simulink model "B2B_MMC"  (R2018b)
settings: Solver=ode8  StartTime=0.0  StopTime=inf  FixedStep=10e-5  RelTol=1e-3
InitFcn:
  | Cd=100e-6;
  | Csm=3.3e-3;
  | L=4e-3;
  | R=0.1;
  | m=1;
  | N=9;
  | Nminus=N-1;
  | 
  | 
  | grid.vll_rms=10e3;
  | grid.f=50;
  | w=2*pi*grid.f;
  | grid.phase=0;
  | grid.va_peak=sqrt(2/3)*grid.vll_rms;
  | 
  | vd_ref=1.05*2*sqrt(2/3)*grid.vll_rms/m; % dc link voltage in pu
  | vsp_max=0.5*m*vd_ref; %phase voltage at phi=0
  | is_max=907;
  | Smax=3*grid.va_peak*is_max/2;
  | 
  | 
  | SCR= 100;  % INPUT SCR of grid at PCC = Ssc_grid/S_rated
  | %Calculated Grid impedance parameters
  | grid.L=grid.va_peak/(w*SCR*is_max); %Calculate Lg out of SRC and neglecting Rg
  | grid.R= w*grid.L/10;        % assume Rg = 10% of Xg [ohm];
  | grid.enable=1;
  | 
  | 
  | 
  | mmc1.load_percent=100;
  | mmc1.load_pf=0.9;
  | 
  | mmc2.load_percent=100;
  | mmc2.load_pf=0.9;
  | 
  | 
  | 
  | mmc1.occ_alpha = 2000;      % INPUT Desired BW output control test converter [rad/s]
  | mmc1.occ_alpha1 = 50;       % INPUT Desired BW of the resonant integrator [rad/s]
  | mmc1.occ_alpha_f = 1000;       % INPUT Desire BW of the VFF [rad/s]
  | 
  | mmc2.occ_alpha = 2000;      % INPUT Desired BW output control test converter [rad/s]
  | mmc2.occ_alpha1 = 50;       % INPUT Desired BW of the resonant integrator [rad/s}
  | mmc2.occ_alpha_f = 1000;       % INPUT Desire BW of the VFF [rad/s
  | 
  | 
  | mmc1.ccc_enable= 1; %INPUT enable ic controller
  | mmc1.ccc_time_enable= 0; %time when circ current control kicks in [s]
  | mmc1.ccc_alpha_cr= 30;  % INPUT BW of LPF for circ current to get the reference (dc value)[rad/s]
  | mmc1.ccc_Ra        = 10;       % INPUT Proportional gain of circ current control (R << Ra < Kp)
  | mmc1.ccc_alpha2 = 200;      % INPUT BW for circulating current test converter  (alpha_c < wgrid)[rad/s]
  | 
  | mmc2.ccc_enable= 1; %INPUT enable ic controller
  | mmc2.ccc_time_enable= 0; %time when circ current control kicks in [s]
  | mmc2.ccc_alpha_cr= 30;  % INPUT BW of LPF for circ current to get the reference (dc value)[rad/s]
  | mmc2.ccc_Ra        = 10;       % INPUT Proportional gain of circ current control (R << Ra < Kp)
  | mmc2.ccc_alpha2 = 200;      % INPUT BW for circulating current test converter  (alpha_c < wgrid)[rad/s]
  | 
  | 
  | mmc1.aec_enable_W= 1; %INPUT enable arm energy controller (Wsum and Wdelta)) at time_W_ctrl
  | mmc1.aec_time_enable_W= 0.8;  % INPUT time to enable W control [s]
  | mmc1.aec_time_Wsum_step = 3;  % INPUT Step time for Sum Energy Step [s]
  | mmc1.aec_WsumRefStep = -0.1;        % INPUT Sum Energy Step at time_SumEn_step [pu]
  | mmc1.aec_enable_Wsum_step  = 1; %INPUT enable Sum Energy step: WsumStep at time: time_WsumRef_step
  | mmc1.aec_alpha_W     = 50;         % INPUT Desired BW for W controler [rad/s]
  | 
  | mmc2.aec_enable_W= 1; %INPUT enable arm energy controller (Wsum and Wdelta)) at time_W_ctrl
  | mmc2.aec_time_enable_W= 0.8;  % INPUT time to enable W control [s]
  | mmc2.aec_time_Wsum_step = 3;  % INPUT Step time for Sum Energy Step [s]
  | mmc2.aec_WsumRefStep = -0.1;        % INPUT Sum Energy Step at time_SumEn_step [pu]
  | mmc2.aec_enable_Wsum_step  = 1; %INPUT enable Sum Energy step: WsumStep at time: time_WsumRef_step
  | mmc2.aec_alpha_W     = 50;         % INPUT Desired BW for W controler [rad/s]
  | 
  | 
  | 
  | mmc1.pll_alpha_b=2000;
  | mmc1.pll_kp=50;
  | mmc1.pll_ki=10;
  | 
  | mmc2.pll_alpha_b=2000;
  | mmc2.pll_kp=50;
  | mmc2.pll_ki=10;
  | 
  | 
  | mmc1.cvdc_alpha_d=50;
  | mmc1.cvdc_alpha_id=25;
  | mmc1.cvdc_enable=1;
  | 
  | mmc2.cvdc_alpha_d=50;
  | mmc2.cvdc_alpha_id=25;
  | mmc2.cvdc_enable=0;
libraries: powerlib x90, powerlib_meascontrol x10, rtlab x1, rtio_opalrt_op5142ex1 x1
(part 1 of 3)
settings Model: Creator=Silov  LastModifiedBy=Silov

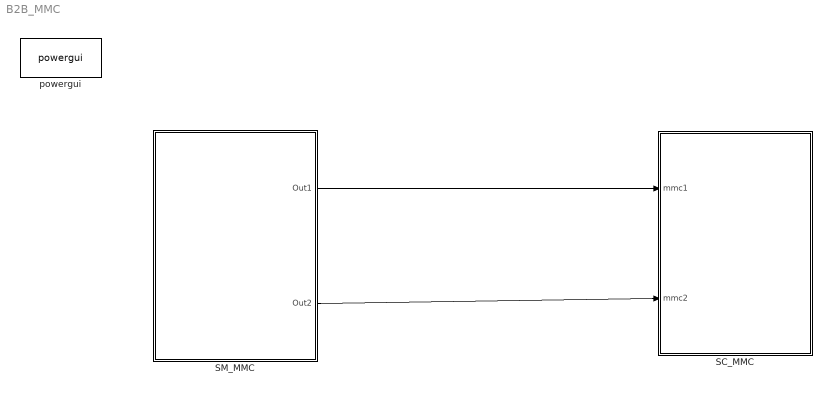
== system B2B_MMC ==
  SC_MMC : Subsystem
  SM_MMC : Subsystem
  powergui : powerlib/powergui  Priority=1  SimulationMode=Discrete  SampleTime=10e-5  frequency=60  Iterations=50  frequencyindice=0  Pbase=100e6  ErrMax=1e-4  UnitsV=kV  UnitsW=MW  buscounter=0  FunctionMessages=off  echomessages=off  EnableUseOfTLC=off  CurrentSourceSwitches=off  DisableSnubberDevices=off  DisableRonSwitches=off  DisableVfSwitches=off  DisplayEquations=off  SolverType=Tustin/Backward Euler (TBE)  Interpol=off  ExternalGateDelay=off  methode=off  Ts=100  x0status=blocks  SPID=on  SwTol=0  HookPort=off  RestoreLinks=warning  ResistiveCurrentMeasurement=off  Frange=[0:2:500]  Ylog=off  Xlog=on  ShowGrid=off  save=off  variable=ZData  structure=0  ZoomFFT=off  StartTime=0.0  cycles=1  DisplayStyle=1  fundamental=60  FreqAxis=off  MaxFrequency=1000  frequencyindicesteady=1  RmsSteady=1  display=off
  wires:
  SM_MMC/1(Out1) -> SC_MMC/1(mmc1)
  SM_MMC/2(Out2) -> SC_MMC/2(mmc2)

== system B2B_MMC/SC_MMC ==
  mmc1 : Inport
  mmc2 : Inport  Port=2
  Active power : Scope  NumInputPorts=2
  Demux : Demux  Outputs=3
  Demux1 : Demux  Outputs=3
  OpComm : rtlab/OpComm  nbport=2  groupe_acq=1  subsys_rate=0  st=0  Synchronization=on  Interpolation=on  Threshold=1.0  Missed_Data=off  Sim_Time=off  Samples=off  dynSigOut=off  from_console=0  warning_done=off  writeOpCommFile=off  Offset=off
  Reactive power : Scope  NumInputPorts=2
  "Voltage " : Scope  NumInputPorts=2
  wires:
  mmc1/1 -> OpComm/1
  mmc2/1 -> OpComm/2
  OpComm/1 -> Demux/1
  OpComm/2 -> Demux1/1
  Demux/1 -> "Voltage "/1
  Demux1/1 -> "Voltage "/2
  Demux/2 -> Active power/1
  Demux1/2 -> Active power/2
  Demux/3 -> Reactive power/1
  Demux1/3 -> Reactive power/2

== system B2B_MMC/SM_MMC ==
  MMC1 : Subsystem
  MMC2 : Subsystem
  OpCtrl OP5142EX1 : rtio_opalrt_op5142ex1/OpCtrl OP5142EX1  CtrlName='OP5142EX1 Ctrl'  boardid=0  BitstreamFilename=OP5142_1-EX-0000-2_2_6_61-16AO_32SelDIO_16AO_32SelDIO-01-01.bin  numconfig=-1  mode=Master  externalClock=off  decimRtsi=0  calibIO=off  SampleTime=0  loadinport=-1
  RSS Grid : Subsystem
  SSS Grid : Subsystem
  dc link impedance : powerlib/Elements/Series RLC Branch  LConnTagsString=__new0  RConnTagsString=__new0  BranchType=RL  Resistance=0.1  Inductance=0.0001  SetiL0=off  InitialCurrent=0  Capacitance=1e-6  Setx0=off  InitialVoltage=0  Measurements=None
  id : powerlib/Measurements/Current Measurement  PhasorSimulation=off  OutputType=Complex  PSBequivalent=0
  meter : powerlib/Measurements/Three-Phase V-I Measurement  VoltageMeasurement=phase-to-ground  SetLabelV=off  LabelV=Vabc  Vpu=off  VpuLL=off  CurrentMeasurement=no  SetLabelI=off  LabelI=Iabc  Ipu=off  Pbase=100e6  Vbase=500e3  OutputType=Complex  PhasorSimulation=off  PSBequivalent=0
  meter1 : powerlib/Measurements/Voltage Measurement  PhasorSimulation=off  OutputType=Complex  PSBequivalent=0
  meter2 : powerlib/Measurements/Three-Phase V-I Measurement  VoltageMeasurement=phase-to-ground  SetLabelV=off  LabelV=Vabc  Vpu=off  VpuLL=off  CurrentMeasurement=no  SetLabelI=off  LabelI=Iabc  Ipu=off  Pbase=100e6  Vbase=500e3  OutputType=Complex  PhasorSimulation=off  PSBequivalent=0
  meter3 : powerlib/Measurements/Voltage Measurement  PhasorSimulation=off  OutputType=Complex  PSBequivalent=0
  Out1 : Outport
  Out2 : Outport  Port=2
  tag scope: rss_vd=global, rss_vpcc=global, sss_id=global, sss_vd=global, sss_vpcc=global
  wires:
  meter1/1 -> [rss_vd]
  MMC1/1(mmc1) -> Out1/1
  meter/1 -> [sss_vpcc]
  meter2/1 -> [rss_vpcc]
  id/1 -> [sss_id]
  meter3/1 -> [sss_vd]
  MMC2/1(mmc2) -> Out2/1
  connections:
  meter1/LConn2 -- meter3/LConn2 -- MMC1/RConn2 -- MMC2/RConn2
  meter/RConn3 -- MMC1/LConn3
  meter/RConn2 -- MMC1/LConn2
  MMC1/RConn1 -- meter3/LConn1 -- id/LConn1
  MMC2/RConn1 -- dc link impedance/RConn1 -- meter1/LConn1
  MMC2/LConn3 -- meter2/RConn3
  meter/LConn2 -- SSS Grid/RConn2
  RSS Grid/RConn1 -- meter2/LConn1
  MMC2/LConn2 -- meter2/RConn2
  meter/RConn1 -- MMC1/LConn1
  meter2/LConn3 -- RSS Grid/RConn3
  MMC2/LConn1 -- meter2/RConn1
  id/RConn1 -- dc link impedance/LConn1
  SSS Grid/RConn3 -- meter/LConn3
  RSS Grid/RConn2 -- meter2/LConn2
  meter/LConn1 -- SSS Grid/RConn1

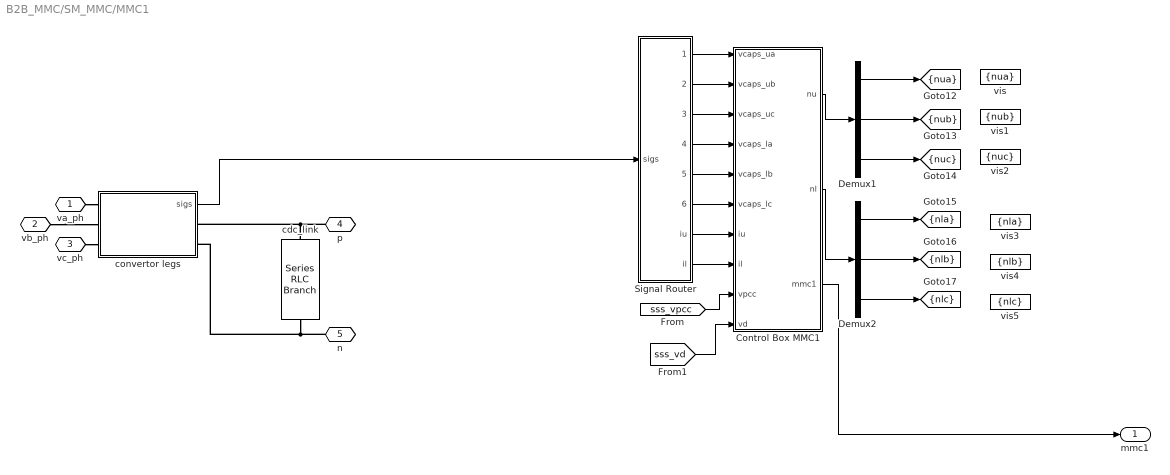
== system B2B_MMC/SM_MMC/MMC1 ==
  Control Box MMC1 : Subsystem  mask{N=N, R=R, L=L, Cd=Cd, Csm=Csm, vd_ref=vd_ref, is_max=is_max, vsp_max=vsp_max, Smax=Smax, occ_alpha=mmc1.occ_alpha, occ_alpha1=mmc1.occ_alpha1, occ_alpha_f=mmc1.occ_alpha_f, ccc_enable=mmc1.ccc_enable, ccc_enable_time=mmc1.ccc_time_enable, ccc_alpha_cr=mmc1.ccc_alpha_cr, ccc_Ra=mmc1.ccc_Ra, ccc_alpha2=mmc1.ccc_alpha2, aec_enable=mmc1.aec_enable_W, aec_enable_time=mmc1.aec_time_enable_W, aec_alpha_W=mmc1.aec_alpha_W, aec_enable_Wsum_step=mmc1.aec_enable_Wsum_step, aec_enable_time_Wsum_step=mmc1.aec_time_Wsum_step, aec_WsumRefStep=mmc1.aec_WsumRefStep, pll_alpha_b=mmc1.pll_alpha_b, pll_kp=mmc1.pll_kp, pll_ki=mmc1.pll_ki, load_percent=mmc1.load_percent, load_pf=mmc1.load_pf, cvdc_enable=mmc1.cvdc_enable, cvdc_alpha_d=mmc1.cvdc_alpha_d, cvdc_alpha_id=mmc1.cvdc_alpha_id}
      mask prompts: N "Number of Submodules"; R "Arm Resistance"; L "Arm Inductance (H)"; Cd "DC Link Capacitance (F)"; Csm "Submodule Capacitance (F)"; vd_ref "DC Link Reference Voltage  (V)"; is_max "Maximum AC Output Current (peak, A)"; vsp_max "Maximum AC Output Voltage (Peak, V)"; Smax "Maximum Apparent Power (VA)"; occ_alpha "Bandwidth, alpha (rad/s)"; occ_alpha1 "Bandwidth, integrator (rad/s)"; occ_alpha_f "Bandwidth for voltage feedforward (rad/s)"; ccc_enable "Enable"; ccc_enable_time "Time of Enable (s)"; ccc_alpha_cr "Bandwidth LPF for DC Reference (rad/s)"; ccc_Ra "Proportional Gain (Ra)"; ccc_alpha2 "Input bandwidth, alpha (rad/s)"; aec_enable "Enable"; aec_enable_time "Enable Time (s)"; aec_alpha_W "Bandwidth (rad/s)"; aec_enable_Wsum_step "Enable Wsum Step"; aec_enable_time_Wsum_step "Enable Wsum Step Time (s)"; aec_WsumRefStep "Step Change in Wsum (p.u.)"; pll_alpha_b "Bandwidth, alpha_b (rad/s)"; pll_kp "Proportional Gain (kp)"; pll_ki "Integral Gain"; load_percent "Percentage Load (%)"; load_pf "Power Factor"; cvdc_enable "Enable"; cvdc_alpha_d "alpha_d"; cvdc_alpha_id "alpha_id"
      mask init:
      | % Output Current Control
      | occ.alpha = occ_alpha;      % INPUT Desired BW output control test converter [rad/s]
      | occ.alpha1= occ_alpha1;       % INPUT Desired BW of the resonant integrator [rad/s}
      | occ.alpha_f = occ_alpha_f;       % INPUT Desire BW of the VFF [rad/s
      | occ.Kp   = occ_alpha*(L/2); % Proportional gain PR conrtoller for output currnet
      | occ.K1   = 2*occ_alpha1*occ.Kp; % Integral gain PI conrtoller for output currnet
      | 
      | % Ciculating current controller
      | ccc.alpha_cr= ccc_alpha_cr;  % INPUT BW of LPF for circ current to get the reference (dc value)[rad/s]
      | ccc.enable_int_ctrl= ccc_enable; %INPUT enable ic controller
      | ccc.time_enable_int_ctrl= ccc_enable_time; %time when circ current control kicks in [s]
      | ccc.Ra        = ccc_Ra;       % INPUT Proportional gain of circ current control (R << Ra < Kp)
      | ccc.alpha2 = ccc_alpha2;      % INPUT BW for circulating current test converter  (alpha_c < wgrid)[rad/s]
      | ccc.K2     = 2*ccc_alpha2;% integral gain for resonant controller for ic for h=2
      | ccc.K1     = ccc.K2;    % integral gain for resonant controller for ic for h=1 (same BW as h=2)
      | ccc.K0     = ccc.K2/10; % integral gain for integrator (alpha0_cc = alfa2_cc/100 << alpha2_cc)
      | 
      | %% Arm Energy Controller
      | aec.enable_W_ctrl= aec_enable; %INPUT enable arm energy controller (Wsum and Wdelta)) at time_W_ctrl
      | aec.time_enable_W_ctrl= aec_enable_time;  % INPUT time to enable W control [s]
      | 
      | WsumRef   = (Csm/N)*vd_ref^2;  % Sum Energy reference [J]
      | aec.alpha_W     = aec_alpha_W;         % INPUT Desired BW for W controler [rad/s]
      | aec.Kp_Wsum     = aec.alpha_W/vd_ref; % Kp*Vd = alpha_Wsum
      | aec.Kp_Wdelta   = aec.alpha_W/vsp_max; % Kp*Vsmax = alpha_Wdelta
      | 
      | aec.time_WsumRef_step = aec_enable_time_Wsum_step;  % INPUT Step time for Sum Energy Step [s]
      | aec.WsumRefStep = aec_WsumRefStep;        % INPUT Sum Energy Step at time_SumEn_step [pu]
      | aec.enable_Wsum_step  = aec_enable_Wsum_step; %INPUT enable Sum Energy step: WsumStep at time: time_WsumRef_step
      | 
      | % PLL Parameters
      | pll.alpha_b=pll_alpha_b;
      | pll.kp=pll_kp;
      | pll.ki=pll_ki;
      | 
      | % Power Control
      | load.percent=load_percent/100;
      | load.phi=acos(load_pf); % It seems that if load.phi is positive then i am injecting reactive power in the grid
      | 
      | % DC Voltage Control variable passes
      | 
      | cvdc.alpha_d=cvdc_alpha_d;
      | cvdc.alpha_id=cvdc_alpha_id;
      | cvdc.enable=cvdc_enable;
      mask DialogControl Parameters Prompt: MMC 1
      mask DialogControl Container7 Prompt: Parameters
      mask DialogControl Design Prompt: Converter Boundaries
      mask DialogControl Container12 Prompt: Current Controllers
      mask DialogControl Container21 Prompt: Output Current
      mask DialogControl Container14 Prompt: Circulating Current
      mask DialogControl Container15 Prompt: Arm Energy
      mask DialogControl Container23 Prompt: Higher Level Control
      mask DialogControl Container22 Prompt: PLL
      mask DialogControl Container20 Prompt: Active and Reactive Powers
      mask DialogControl Container9 Prompt: DC Voltage Control
  Demux1 : Demux  Outputs=3
  Demux2 : Demux  Outputs=3
  Signal Router : Subsystem
  cdc_link : powerlib/Elements/Series RLC Branch  LConnTagsString=__new0  RConnTagsString=__new0  BranchType=C  Resistance=1  Inductance=1e-3  SetiL0=off  InitialCurrent=0  Capacitance=Cd  Setx0=on  InitialVoltage=vd_ref  Measurements=None
  convertor legs : Subsystem
  vis : GotoTagVisibility  GotoTag=nua
  vis1 : GotoTagVisibility  GotoTag=nub
  vis2 : GotoTagVisibility  GotoTag=nuc
  vis3 : GotoTagVisibility  GotoTag=nla
  vis4 : GotoTagVisibility  GotoTag=nlb
  vis5 : GotoTagVisibility  GotoTag=nlc
  va_ph : PMIOPort  Side=Left
  vb_ph : PMIOPort  Port=2  Side=Left
  vc_ph : PMIOPort  Port=3  Side=Left
  p : PMIOPort  Port=4  Side=Right
  n : PMIOPort  Port=5  Side=Right
  mmc1 : Outport
  tag scope: nla=scoped, nlb=scoped, nlc=scoped, nua=scoped, nub=scoped, nuc=scoped
  wires:
  convertor legs/1(sigs) -> Signal Router/1(sigs)
  Signal Router/1(vc_ua) -> Control Box MMC1/1(vcaps_ua)
  Signal Router/2(vc_ub) -> Control Box MMC1/2(vcaps_ub)
  Signal Router/3(vc_uc) -> Control Box MMC1/3(vcaps_uc)
  Signal Router/4(vc_la) -> Control Box MMC1/4(vcaps_la)
  Signal Router/5(vc_lb) -> Control Box MMC1/5(vcaps_lb)
  Signal Router/6(vc_lc) -> Control Box MMC1/6(vcaps_lc)
  Signal Router/7(iu) -> Control Box MMC1/7(iu)
  Signal Router/8(il) -> Control Box MMC1/8(il)
  Demux2/1 -> [nla]
  Demux2/3 -> [nlc]
  Demux2/2 -> [nlb]
  Control Box MMC1/2(nl) -> Demux2/1
  Demux1/1 -> [nua]
  Demux1/3 -> [nuc]
  Demux1/2 -> [nub]
  Control Box MMC1/1(nu) -> Demux1/1
  [sss_vpcc] -> Control Box MMC1/9(vpcc)
  [sss_vd] -> Control Box MMC1/10(vd)
  Control Box MMC1/3(mmc1) -> mmc1/1
  connections:
  cdc_link/LConn1 -- p/RConn1 -- convertor legs/RConn1
  cdc_link/RConn1 -- n/RConn1 -- convertor legs/RConn2
  va_ph/RConn1 -- convertor legs/LConn1
  vb_ph/RConn1 -- convertor legs/LConn2
  vc_ph/RConn1 -- convertor legs/LConn3

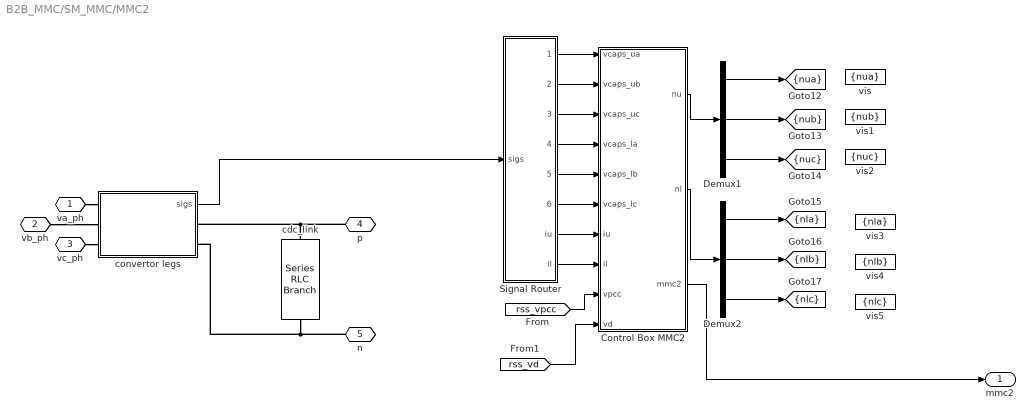
== system B2B_MMC/SM_MMC/MMC2 ==
  Control Box MMC2 : Subsystem  mask{N=N, R=R, L=L, Cd=Cd, Csm=Csm, vd_ref=vd_ref, is_max=is_max, vsp_max=vsp_max, Smax=Smax, occ_alpha=mmc2.occ_alpha, occ_alpha1=mmc2.occ_alpha1, occ_alpha_f=mmc2.occ_alpha_f, ccc_enable=mmc2.ccc_enable, ccc_enable_time=mmc2.ccc_time_enable, ccc_alpha_cr=mmc2.ccc_alpha_cr, ccc_Ra=mmc2.ccc_Ra, ccc_alpha2=mmc2.ccc_alpha2, aec_enable=mmc2.aec_enable_W, aec_enable_time=mmc2.aec_time_enable_W, aec_alpha_W=mmc2.aec_alpha_W, aec_enable_Wsum_step=mmc2.aec_enable_Wsum_step, aec_enable_time_Wsum_step=mmc2.aec_time_Wsum_step, aec_WsumRefStep=mmc2.aec_WsumRefStep, pll_alpha_b=mmc2.pll_alpha_b, pll_kp=mmc2.pll_kp, pll_ki=mmc2.pll_ki, load_percent=mmc2.load_percent, load_pf=mmc2.load_pf, cvdc_enable=mmc2.cvdc_enable, cvdc_alpha_d=mmc2.cvdc_alpha_d, cvdc_alpha_id=mmc2.cvdc_alpha_id}
      mask prompts: N "Number of Submodules"; R "Arm Resistance"; L "Arm Inductance (H)"; Cd "DC Link Capacitance (F)"; Csm "Submodule Capacitance (F)"; vd_ref "DC Link Reference Voltage  (V)"; is_max "Maximum AC Output Current (peak, A)"; vsp_max "Maximum AC Output Voltage (Peak, V)"; Smax "Maximum Apparent Power (VA)"; occ_alpha "Bandwidth, alpha (rad/s)"; occ_alpha1 "Bandwidth, integrator (rad/s)"; occ_alpha_f "Bandwidth for voltage feedforward (rad/s)"; ccc_enable "Enable"; ccc_enable_time "Time of Enable (s)"; ccc_alpha_cr "Bandwidth LPF for DC Reference (rad/s)"; ccc_Ra "Proportional Gain (Ra)"; ccc_alpha2 "Input bandwidth, alpha (rad/s)"; aec_enable "Enable"; aec_enable_time "Enable Time (s)"; aec_alpha_W "Bandwidth (rad/s)"; aec_enable_Wsum_step "Enable Wsum Step"; aec_enable_time_Wsum_step "Enable Wsum Step Time (s)"; aec_WsumRefStep "Step Change in Wsum (p.u.)"; pll_alpha_b "Bandwidth, alpha_b (rad/s)"; pll_kp "Proportional Gain (kp)"; pll_ki "Integral Gain"; load_percent "Percentage Load (%)"; load_pf "Power Factor"; cvdc_enable "Enable"; cvdc_alpha_d "alpha_d"; cvdc_alpha_id "alpha_id"
      mask init: same as B2B_MMC/SM_MMC/MMC1/Control Box MMC1
      mask DialogControl Parameters Prompt: MMC 1
      mask DialogControl Container7 Prompt: Parameters
      mask DialogControl Design Prompt: Converter Boundaries
      mask DialogControl Container12 Prompt: Current Controllers
      mask DialogControl Container21 Prompt: Output Current
      mask DialogControl Container14 Prompt: Circulating Current
      mask DialogControl Container15 Prompt: Arm Energy
      mask DialogControl Container23 Prompt: Higher Level Control
      mask DialogControl Container22 Prompt: PLL
      mask DialogControl Container20 Prompt: Active and Reactive Powers
      mask DialogControl Container9 Prompt: DC Voltage Control
  Demux1 : Demux  Outputs=3
  Demux2 : Demux  Outputs=3
  Signal Router : Subsystem
  cdc_link : powerlib/Elements/Series RLC Branch  LConnTagsString=__new0  RConnTagsString=__new0  BranchType=C  Resistance=1  Inductance=1e-3  SetiL0=off  InitialCurrent=0  Capacitance=Cd  Setx0=on  InitialVoltage=vd_ref  Measurements=None
  convertor legs : Subsystem
  vis : GotoTagVisibility  GotoTag=nua
  vis1 : GotoTagVisibility  GotoTag=nub
  vis2 : GotoTagVisibility  GotoTag=nuc
  vis3 : GotoTagVisibility  GotoTag=nla
  vis4 : GotoTagVisibility  GotoTag=nlb
  vis5 : GotoTagVisibility  GotoTag=nlc
  va_ph : PMIOPort  Side=Left
  vb_ph : PMIOPort  Port=2  Side=Left
  vc_ph : PMIOPort  Port=3  Side=Left
  p : PMIOPort  Port=4  Side=Right
  n : PMIOPort  Port=5  Side=Right
  mmc2 : Outport
  tag scope: nla=scoped, nlb=scoped, nlc=scoped, nua=scoped, nub=scoped, nuc=scoped
  wires:
  convertor legs/1(sigs) -> Signal Router/1(sigs)
  Signal Router/1(vc_ua) -> Control Box MMC2/1(vcaps_ua)
  Signal Router/2(vc_ub) -> Control Box MMC2/2(vcaps_ub)
  Signal Router/3(vc_uc) -> Control Box MMC2/3(vcaps_uc)
  Signal Router/4(vc_la) -> Control Box MMC2/4(vcaps_la)
  Signal Router/5(vc_lb) -> Control Box MMC2/5(vcaps_lb)
  Signal Router/6(vc_lc) -> Control Box MMC2/6(vcaps_lc)
  Signal Router/7(iu) -> Control Box MMC2/7(iu)
  Signal Router/8(il) -> Control Box MMC2/8(il)
  Demux2/1 -> [nla]
  Demux2/3 -> [nlc]
  Demux2/2 -> [nlb]
  Control Box MMC2/2(nl) -> Demux2/1
  Demux1/1 -> [nua]
  Demux1/3 -> [nuc]
  Demux1/2 -> [nub]
  Control Box MMC2/1(nu) -> Demux1/1
  [rss_vpcc] -> Control Box MMC2/9(vpcc)
  [rss_vd] -> Control Box MMC2/10(vd)
  Control Box MMC2/3(mmc2) -> mmc2/1
  connections:
  cdc_link/LConn1 -- convertor legs/RConn1 -- p/RConn1
  cdc_link/RConn1 -- convertor legs/RConn2 -- n/RConn1
  va_ph/RConn1 -- convertor legs/LConn1
  vb_ph/RConn1 -- convertor legs/LConn2
  vc_ph/RConn1 -- convertor legs/LConn3

== system B2B_MMC/SM_MMC/RSS Grid ==
  Three-Phase Series RLC Branch : powerlib/Elements/Three-Phase Series RLC Branch  LConnTagsString=A|B|C  RConnTagsString=A|B|C  BranchType=RL  Resistance=grid.R  Inductance=grid.L  Capacitance=1e-6  Measurements=None
  grid voltage : Subsystem
  va_ph : PMIOPort  Side=Right
  vb_ph : PMIOPort  Port=2  Side=Right
  vc_ph : PMIOPort  Port=3  Side=Right
  connections:
  grid voltage/RConn1 -- Three-Phase Series RLC Branch/LConn1
  grid voltage/RConn2 -- Three-Phase Series RLC Branch/LConn2
  grid voltage/RConn3 -- Three-Phase Series RLC Branch/LConn3
  va_ph/RConn1 -- Three-Phase Series RLC Branch/RConn1
  Three-Phase Series RLC Branch/RConn2 -- vb_ph/RConn1
  vc_ph/RConn1 -- Three-Phase Series RLC Branch/RConn3

== system B2B_MMC/SM_MMC/SSS Grid ==
  Three-Phase Series RLC Branch : powerlib/Elements/Three-Phase Series RLC Branch  LConnTagsString=A|B|C  RConnTagsString=A|B|C  BranchType=RL  Resistance=grid.R  Inductance=grid.L  Capacitance=1e-6  Measurements=None
  grid voltage : Subsystem
  va_ph : PMIOPort  Side=Right
  vb_ph : PMIOPort  Port=2  Side=Right
  vc_ph : PMIOPort  Port=3  Side=Right
  connections:
  grid voltage/RConn1 -- Three-Phase Series RLC Branch/LConn1
  grid voltage/RConn2 -- Three-Phase Series RLC Branch/LConn2
  grid voltage/RConn3 -- Three-Phase Series RLC Branch/LConn3
  va_ph/RConn1 -- Three-Phase Series RLC Branch/RConn1
  Three-Phase Series RLC Branch/RConn2 -- vb_ph/RConn1
  vc_ph/RConn1 -- Three-Phase Series RLC Branch/RConn3

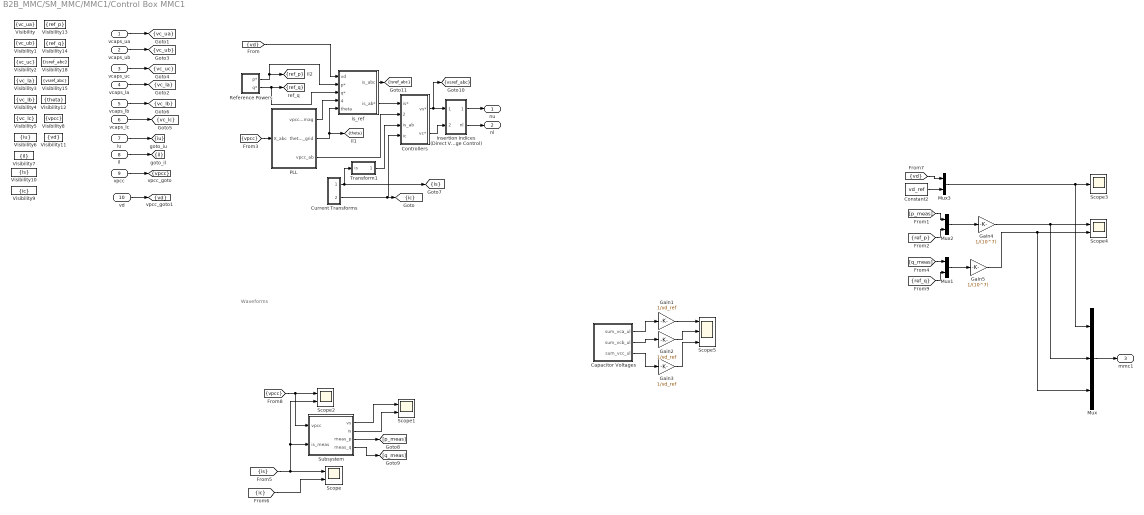
== system B2B_MMC/SM_MMC/MMC1/Control Box MMC1 ==
  note: Waveforms
  vcaps_ua : Inport
  vcaps_ub : Inport  Port=2
  vcaps_uc : Inport  Port=3
  vcaps_la : Inport  Port=4
  vcaps_lb : Inport  Port=5
  vcaps_lc : Inport  Port=6
  iu : Inport  Port=7
  il : Inport  Port=8
  vpcc : Inport  Port=9
  vd : Inport  Port=10
  Capacitor Voltages : Subsystem
  Constant2 : Constant  Value=vd_ref
  Controllers : Subsystem
  Current Transforms : Subsystem
  Gain1 : Gain  Gain=1/vd_ref
  Gain2 : Gain  Gain=1/vd_ref
  Gain3 : Gain  Gain=1/vd_ref
  Gain4 : Gain  Gain=1/(10^7)
  Gain5 : Gain  Gain=1/(10^7)
  Insertion Indices (Direct Voltage Control) : Subsystem
  Mux : Mux  Inputs=3
  Mux1 : Mux  Inputs=2
  Mux2 : Mux  Inputs=2
  Mux3 : Mux  Inputs=2
  PLL : Subsystem
  Reference Powers : Subsystem
  Scope{,1..2,4} (4 alike) : Scope  NumInputPorts=2
  Scope3 : Scope
  Scope5 : Scope  NumInputPorts=3
  Subsystem : Subsystem
  Transform1 : Subsystem
  Visibility : GotoTagVisibility  GotoTag=vc_ua
  Visibility1 : GotoTagVisibility  GotoTag=vc_ub
  Visibility10 : GotoTagVisibility  GotoTag=is
  Visibility11 : GotoTagVisibility  GotoTag=vd
  Visibility12 : GotoTagVisibility  GotoTag=theta
  Visibility13 : GotoTagVisibility  GotoTag=ref_p
  Visibility14 : GotoTagVisibility  GotoTag=ref_q
  Visibility15 : GotoTagVisibility  GotoTag=vsref_abc
  Visibility18 : GotoTagVisibility  GotoTag=isref_abc
  Visibility2 : GotoTagVisibility  GotoTag=vc_uc
  Visibility3 : GotoTagVisibility  GotoTag=vc_la
  Visibility4 : GotoTagVisibility  GotoTag=vc_lb
  Visibility5 : GotoTagVisibility  GotoTag=vc_lc
  Visibility6 : GotoTagVisibility  GotoTag=iu
  Visibility7 : GotoTagVisibility  GotoTag=il
  Visibility8 : GotoTagVisibility  GotoTag=vpcc
  Visibility9 : GotoTagVisibility  GotoTag=ic
  is_ref : Subsystem
  nu : Outport
  nl : Outport  Port=2
  mmc1 : Outport  Port=3
  tag scope: ic=scoped, il=scoped, is=scoped, isref_abc=scoped, iu=scoped, ref_p=scoped, ref_q=scoped, theta=scoped, vc_la=scoped, vc_lb=scoped, vc_lc=scoped, vc_ua=scoped, vc_ub=scoped, vc_uc=scoped, vd=scoped, vpcc=scoped, vsref_abc=scoped
  wires:
  Controllers/2(vc*) -> Insertion Indices (Direct Voltage Control)/2(vc*)
  Current Transforms/1(is) -> [is], Transform1/1(is)
  Reference Powers/2(q*) -> is_ref/3(q*), [ref_q]
  Transform1/1(is_ab) -> Controllers/3(is_ab)
  Controllers/1(vs*) -> [vsref_abc], Insertion Indices (Direct Voltage Control)/1(vs*)
  PLL/3(vpcc_ab) -> Controllers/2(vpcc_ab)
  is_ref/2(is_ab*) -> Controllers/1(is*)
  Current Transforms/2(ic) -> Controllers/4(ic), [ic]
  [vpcc] -> PLL/1(X_abc)
  is_ref/1(is_abc) -> [isref_abc]
  Reference Powers/1(p*) -> is_ref/2(p*), [ref_p]
  PLL/2(theta_grid) -> is_ref/5(theta), [theta]
  PLL/1(vpcc_mag) -> is_ref/4(vpll_mag)
  vcaps_ua/1 -> [vc_ua]
  vcaps_ub/1 -> [vc_ub]
  vcaps_uc/1 -> [vc_uc]
  iu/1 -> [iu]
  il/1 -> [il]
  vpcc/1 -> [vpcc]
  vcaps_la/1 -> [vc_la]
  vcaps_lb/1 -> [vc_lb]
  vcaps_lc/1 -> [vc_lc]
  Insertion Indices (Direct Voltage Control)/1(nu) -> nu/1
  Insertion Indices (Direct Voltage Control)/2(nl) -> nl/1
  vd/1 -> [vd]
  [vd] -> is_ref/1(vd)
  Mux3/1 -> Mux/1, Scope3/1
  Constant2/1 -> Mux3/2
  [vd] -> Mux3/1
  Subsystem/4(meas_q) -> [q_meas]
  Subsystem/3(meas_p) -> [p_meas]
  [is] -> Scope/1, Scope2/2, Subsystem/2(is_meas)
  [ic] -> Scope/2
  Capacitor Voltages/3(sum_vcc_ul) -> Gain3/1
  Capacitor Voltages/2(sum_vcb_ul) -> Gain2/1
  Capacitor Voltages/1(sum_vca_ul) -> Gain1/1
  Gain1/1 -> Scope5/1
  Gain2/1 -> Scope5/2
  Gain3/1 -> Scope5/3
  Gain5/1 -> Mux/3, Scope4/2
  Mux1/1 -> Gain5/1
  Gain4/1 -> Mux/2, Scope4/1
  Mux2/1 -> Gain4/1
  [q_meas] -> Mux1/1
  [ref_q] -> Mux1/2
  [p_meas] -> Mux2/1
  [ref_p] -> Mux2/2
  Subsystem/2(is) -> Scope1/2
  Subsystem/1(vs) -> Scope1/1
  [vpcc] -> Scope2/1, Subsystem/1(vpcc)
  Mux/1 -> mmc1/1

== system B2B_MMC/SM_MMC/MMC1/Signal Router ==
  sigs : Inport
  Demux : Demux  Outputs=12
  Mux : Mux  Inputs=3
  Mux1 : Mux  Inputs=3
  vc_ua : Outport
  vc_ub : Outport  Port=2
  vc_uc : Outport  Port=3
  vc_la : Outport  Port=4
  vc_lb : Outport  Port=5
  vc_lc : Outport  Port=6
  iu : Outport  Port=7
  il : Outport  Port=8
  wires:
  Demux/9 -> vc_uc/1
  Demux/1 -> Mux/1
  Demux/8 -> vc_ub/1
  Demux/7 -> vc_ua/1
  Demux/12 -> vc_lc/1
  Demux/3 -> Mux/3
  Demux/6 -> Mux1/3
  Demux/5 -> Mux1/2
  Mux1/1 -> il/1
  Demux/4 -> Mux1/1
  Demux/11 -> vc_lb/1
  sigs/1 -> Demux/1
  Mux/1 -> iu/1
  Demux/2 -> Mux/2
  Demux/10 -> vc_la/1

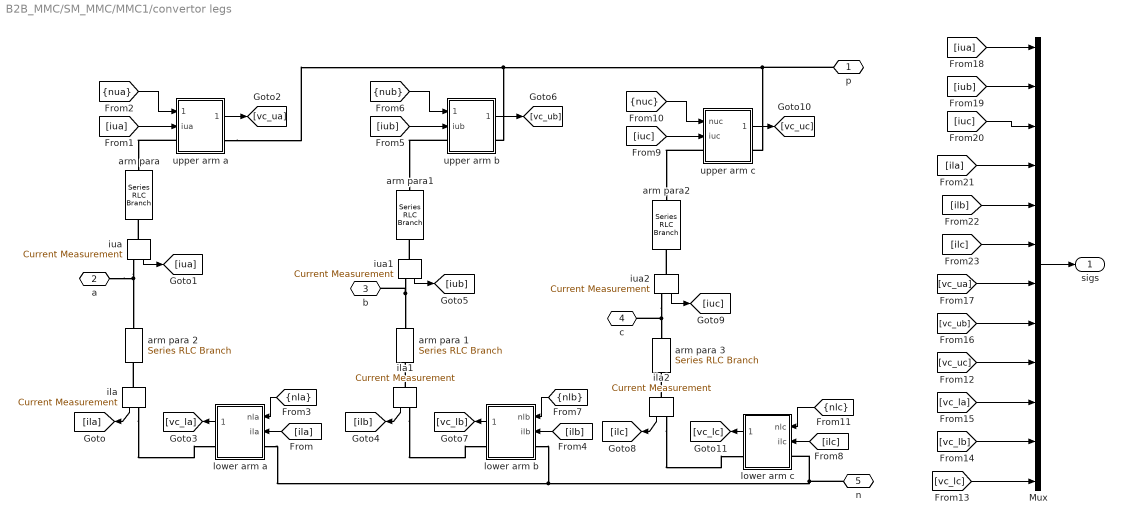
== system B2B_MMC/SM_MMC/MMC1/convertor legs ==
  Mux : Mux  Inputs=12
  arm para : powerlib/Elements/Series RLC Branch  LConnTagsString=__new0  RConnTagsString=__new0  BranchType=RL  Resistance=R  Inductance=L  SetiL0=off  InitialCurrent=0  Capacitance=1e-6  Setx0=off  InitialVoltage=0  Measurements=None
  arm para 1 : powerlib/Elements/Series RLC Branch  LConnTagsString=__new0  RConnTagsString=__new0  BranchType=RL  Resistance=R  Inductance=L  SetiL0=off  InitialCurrent=0  Capacitance=1e-6  Setx0=off  InitialVoltage=0  Measurements=None
  arm para 2 : powerlib/Elements/Series RLC Branch  LConnTagsString=__new0  RConnTagsString=__new0  BranchType=RL  Resistance=R  Inductance=L  SetiL0=off  InitialCurrent=0  Capacitance=1e-6  Setx0=off  InitialVoltage=0  Measurements=None
  arm para 3 : powerlib/Elements/Series RLC Branch  LConnTagsString=__new0  RConnTagsString=__new0  BranchType=RL  Resistance=R  Inductance=L  SetiL0=off  InitialCurrent=0  Capacitance=1e-6  Setx0=off  InitialVoltage=0  Measurements=None
  arm para1 : powerlib/Elements/Series RLC Branch  LConnTagsString=__new0  RConnTagsString=__new0  BranchType=RL  Resistance=R  Inductance=L  SetiL0=off  InitialCurrent=0  Capacitance=1e-6  Setx0=off  InitialVoltage=0  Measurements=None
  arm para2 : powerlib/Elements/Series RLC Branch  LConnTagsString=__new0  RConnTagsString=__new0  BranchType=RL  Resistance=R  Inductance=L  SetiL0=off  InitialCurrent=0  Capacitance=1e-6  Setx0=off  InitialVoltage=0  Measurements=None
  ila : powerlib/Measurements/Current Measurement  PhasorSimulation=off  OutputType=Complex  PSBequivalent=0
  ila1 : powerlib/Measurements/Current Measurement  PhasorSimulation=off  OutputType=Complex  PSBequivalent=0
  ila2 : powerlib/Measurements/Current Measurement  PhasorSimulation=off  OutputType=Complex  PSBequivalent=0
  iua : powerlib/Measurements/Current Measurement  PhasorSimulation=off  OutputType=Complex  PSBequivalent=0
  iua1 : powerlib/Measurements/Current Measurement  PhasorSimulation=off  OutputType=Complex  PSBequivalent=0
  iua2 : powerlib/Measurements/Current Measurement  PhasorSimulation=off  OutputType=Complex  PSBequivalent=0
  lower arm a : Subsystem
  lower arm b : Subsystem
  lower arm c : Subsystem
  upper arm a : Subsystem
  upper arm b : Subsystem
  upper arm c : Subsystem
  p : PMIOPort  Side=Right
  a : PMIOPort  Port=2  Side=Left
  b : PMIOPort  Port=3  Side=Left
  c : PMIOPort  Port=4  Side=Left
  n : PMIOPort  Port=5  Side=Right
  sigs : Outport
  wires:
  lower arm b/1(vc_lb) -> [vc_lb]
  iua1/1 -> [iub]
  [nlb] -> lower arm b/1(nlb)
  ila/1 -> [ila]
  iua/1 -> [iua]
  [ila] -> lower arm a/2(ila)
  upper arm a/1(vc_ua) -> [vc_ua]
  lower arm a/1(vc_la) -> [vc_la]
  [ilb] -> lower arm b/2(ilb)
  [iua] -> upper arm a/2(iua)
  [nua] -> upper arm a/1(nua)
  [nub] -> upper arm b/1(nub)
  ila1/1 -> [ilb]
  [iub] -> upper arm b/2(iub)
  [nla] -> lower arm a/1(nla)
  upper arm b/1(vc_ub) -> [vc_ub]
  lower arm c/1(vc_lc) -> [vc_lc]
  [nlc] -> lower arm c/1(nlc)
  [iuc] -> upper arm c/2(iuc)
  [ilc] -> lower arm c/2(ilc)
  [nuc] -> upper arm c/1(nuc)
  ila2/1 -> [ilc]
  iua2/1 -> [iuc]
  upper arm c/1(vc_uc) -> [vc_uc]
  [vc_lc] -> Mux/12
  [vc_lb] -> Mux/11
  [vc_la] -> Mux/10
  [vc_uc] -> Mux/9
  [vc_ub] -> Mux/8
  [vc_ua] -> Mux/7
  [iua] -> Mux/1
  [iub] -> Mux/2
  [iuc] -> Mux/3
  [ila] -> Mux/4
  [ilb] -> Mux/5
  [ilc] -> Mux/6
  Mux/1 -> sigs/1
  connections:
  upper arm b/LConn1 -- arm para1/LConn1
  ila/RConn1 -- lower arm a/RConn1
  ila/LConn1 -- arm para 2/RConn1
  ila1/LConn1 -- arm para 1/RConn1
  iua/RConn1 -- a/RConn1 -- arm para 2/LConn1
  iua1/RConn1 -- b/RConn1 -- arm para 1/LConn1
  iua1/LConn1 -- arm para1/RConn1
  ila1/RConn1 -- lower arm b/RConn1
  iua/LConn1 -- arm para/RConn1
  upper arm a/LConn1 -- arm para/LConn1
  ila2/RConn1 -- lower arm c/RConn1
  iua2/LConn1 -- arm para2/RConn1
  iua2/RConn1 -- c/RConn1 -- arm para 3/LConn1
  upper arm c/LConn1 -- arm para2/LConn1
  ila2/LConn1 -- arm para 3/RConn1
  lower arm b/LConn1 -- lower arm a/LConn1 -- n/RConn1 -- lower arm c/LConn1
  upper arm a/RConn1 -- upper arm b/RConn1 -- upper arm c/RConn1 -- p/RConn1

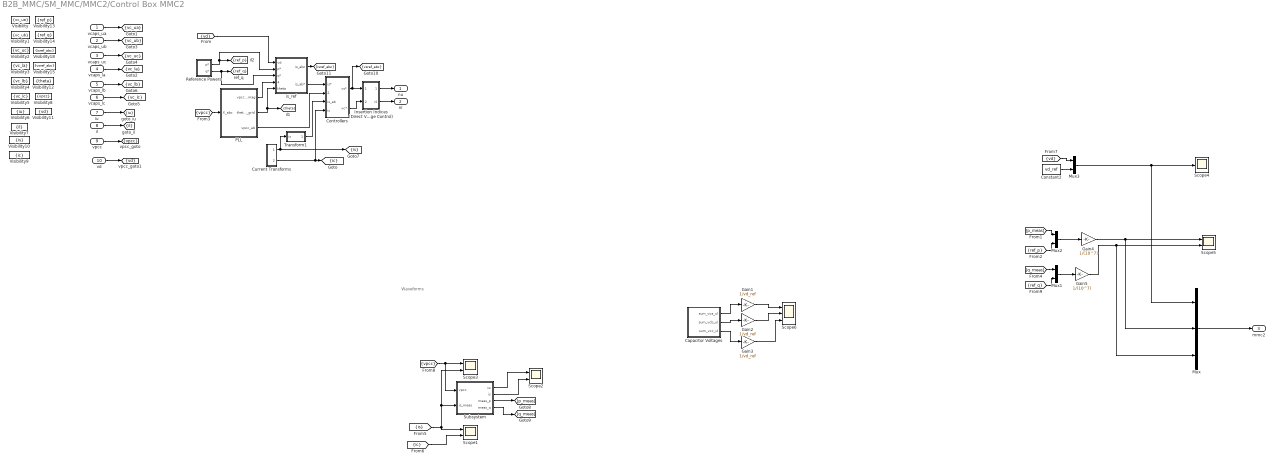
== system B2B_MMC/SM_MMC/MMC2/Control Box MMC2 ==
  note: Waveforms
  vcaps_ua : Inport
  vcaps_ub : Inport  Port=2
  vcaps_uc : Inport  Port=3
  vcaps_la : Inport  Port=4
  vcaps_lb : Inport  Port=5
  vcaps_lc : Inport  Port=6
  iu : Inport  Port=7
  il : Inport  Port=8
  vpcc : Inport  Port=9
  vd : Inport  Port=10
  Capacitor Voltages : Subsystem
  Constant2 : Constant  Value=vd_ref
  Controllers : Subsystem
  Current Transforms : Subsystem
  Gain1 : Gain  Gain=1/vd_ref
  Gain2 : Gain  Gain=1/vd_ref
  Gain3 : Gain  Gain=1/vd_ref
  Gain4 : Gain  Gain=1/(10^7)
  Gain5 : Gain  Gain=1/(10^7)
  Insertion Indices (Direct Voltage Control) : Subsystem
  Mux : Mux  Inputs=3
  Mux1 : Mux  Inputs=2
  Mux2 : Mux  Inputs=2
  Mux3 : Mux  Inputs=2
  PLL : Subsystem
  Reference Powers : Subsystem
  Scope{1..3,5} (4 alike) : Scope  NumInputPorts=2
  Scope4 : Scope
  Scope6 : Scope  NumInputPorts=3
  Subsystem : Subsystem
  Transform1 : Subsystem
  Visibility : GotoTagVisibility  GotoTag=vc_ua
  Visibility1 : GotoTagVisibility  GotoTag=vc_ub
  Visibility10 : GotoTagVisibility  GotoTag=is
  Visibility11 : GotoTagVisibility  GotoTag=vd
  Visibility12 : GotoTagVisibility  GotoTag=theta
  Visibility13 : GotoTagVisibility  GotoTag=ref_p
  Visibility14 : GotoTagVisibility  GotoTag=ref_q
  Visibility15 : GotoTagVisibility  GotoTag=vsref_abc
  Visibility18 : GotoTagVisibility  GotoTag=isref_abc
  Visibility2 : GotoTagVisibility  GotoTag=vc_uc
  Visibility3 : GotoTagVisibility  GotoTag=vc_la
  Visibility4 : GotoTagVisibility  GotoTag=vc_lb
  Visibility5 : GotoTagVisibility  GotoTag=vc_lc
  Visibility6 : GotoTagVisibility  GotoTag=iu
  Visibility7 : GotoTagVisibility  GotoTag=il
  Visibility8 : GotoTagVisibility  GotoTag=vpcc
  Visibility9 : GotoTagVisibility  GotoTag=ic
  is_ref : Subsystem
  nu : Outport
  nl : Outport  Port=2
  mmc2 : Outport  Port=3
  tag scope: ic=scoped, il=scoped, is=scoped, isref_abc=scoped, iu=scoped, ref_p=scoped, ref_q=scoped, theta=scoped, vc_la=scoped, vc_lb=scoped, vc_lc=scoped, vc_ua=scoped, vc_ub=scoped, vc_uc=scoped, vd=scoped, vpcc=scoped, vsref_abc=scoped
  wires:
  Controllers/2(vc*) -> Insertion Indices (Direct Voltage Control)/2(vc*)
  Current Transforms/1(is) -> [is], Transform1/1(is)
  Reference Powers/2(q*) -> is_ref/3(q*), [ref_q]
  Transform1/1(is_ab) -> Controllers/3(is_ab)
  Controllers/1(vs*) -> [vsref_abc], Insertion Indices (Direct Voltage Control)/1(vs*)
  PLL/3(vpcc_ab) -> Controllers/2(vpcc_ab)
  is_ref/2(is_ab*) -> Controllers/1(is*)
  Current Transforms/2(ic) -> Controllers/4(ic), [ic]
  [vpcc] -> PLL/1(X_abc)
  is_ref/1(is_abc) -> [isref_abc]
  Reference Powers/1(p*) -> is_ref/2(p*), [ref_p]
  PLL/2(theta_grid) -> is_ref/5(theta), [theta]
  PLL/1(vpcc_mag) -> is_ref/4(vpll_mag)
  vcaps_ua/1 -> [vc_ua]
  vcaps_ub/1 -> [vc_ub]
  vcaps_uc/1 -> [vc_uc]
  iu/1 -> [iu]
  il/1 -> [il]
  vpcc/1 -> [vpcc]
  vcaps_la/1 -> [vc_la]
  vcaps_lb/1 -> [vc_lb]
  vcaps_lc/1 -> [vc_lc]
  Insertion Indices (Direct Voltage Control)/1(nu) -> nu/1
  Insertion Indices (Direct Voltage Control)/2(nl) -> nl/1
  vd/1 -> [vd]
  [vd] -> is_ref/1(vd)
  Mux3/1 -> Mux/1, Scope4/1
  Constant2/1 -> Mux3/2
  [vd] -> Mux3/1
  Subsystem/4(meas_q) -> [q_meas]
  Subsystem/3(meas_p) -> [p_meas]
  [is] -> Scope1/1, Scope3/2, Subsystem/2(is_meas)
  [ic] -> Scope1/2
  Capacitor Voltages/3(sum_vcc_ul) -> Gain3/1
  Capacitor Voltages/2(sum_vcb_ul) -> Gain2/1
  Capacitor Voltages/1(sum_vca_ul) -> Gain1/1
  Gain1/1 -> Scope6/1
  Gain2/1 -> Scope6/2
  Gain3/1 -> Scope6/3
  Gain5/1 -> Mux/3, Scope5/2
  Mux1/1 -> Gain5/1
  Gain4/1 -> Mux/2, Scope5/1
  Mux2/1 -> Gain4/1
  [q_meas] -> Mux1/1
  [ref_q] -> Mux1/2
  [p_meas] -> Mux2/1
  [ref_p] -> Mux2/2
  Subsystem/2(is) -> Scope2/2
  Subsystem/1(vs) -> Scope2/1
  [vpcc] -> Scope3/1, Subsystem/1(vpcc)
  Mux/1 -> mmc2/1

== system B2B_MMC/SM_MMC/MMC2/Signal Router ==
  sigs : Inport
  Demux : Demux  Outputs=12
  Mux : Mux  Inputs=3
  Mux1 : Mux  Inputs=3
  vc_ua : Outport
  vc_ub : Outport  Port=2
  vc_uc : Outport  Port=3
  vc_la : Outport  Port=4
  vc_lb : Outport  Port=5
  vc_lc : Outport  Port=6
  iu : Outport  Port=7
  il : Outport  Port=8
  wires:
  Demux/9 -> vc_uc/1
  Demux/1 -> Mux/1
  Demux/8 -> vc_ub/1
  Demux/7 -> vc_ua/1
  Demux/12 -> vc_lc/1
  Demux/3 -> Mux/3
  Demux/6 -> Mux1/3
  Demux/5 -> Mux1/2
  Mux1/1 -> il/1
  Demux/4 -> Mux1/1
  Demux/11 -> vc_lb/1
  sigs/1 -> Demux/1
  Mux/1 -> iu/1
  Demux/2 -> Mux/2
  Demux/10 -> vc_la/1

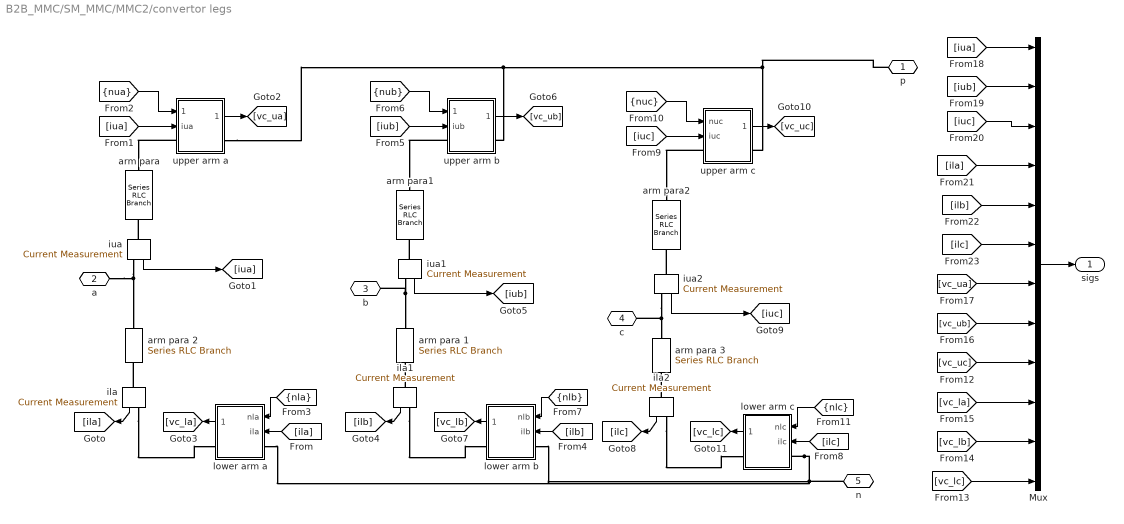
== system B2B_MMC/SM_MMC/MMC2/convertor legs ==
  Mux : Mux  Inputs=12
  arm para : powerlib/Elements/Series RLC Branch  LConnTagsString=__new0  RConnTagsString=__new0  BranchType=RL  Resistance=R  Inductance=L  SetiL0=off  InitialCurrent=0  Capacitance=1e-6  Setx0=off  InitialVoltage=0  Measurements=None
  arm para 1 : powerlib/Elements/Series RLC Branch  LConnTagsString=__new0  RConnTagsString=__new0  BranchType=RL  Resistance=R  Inductance=L  SetiL0=off  InitialCurrent=0  Capacitance=1e-6  Setx0=off  InitialVoltage=0  Measurements=None
  arm para 2 : powerlib/Elements/Series RLC Branch  LConnTagsString=__new0  RConnTagsString=__new0  BranchType=RL  Resistance=R  Inductance=L  SetiL0=off  InitialCurrent=0  Capacitance=1e-6  Setx0=off  InitialVoltage=0  Measurements=None
  arm para 3 : powerlib/Elements/Series RLC Branch  LConnTagsString=__new0  RConnTagsString=__new0  BranchType=RL  Resistance=R  Inductance=L  SetiL0=off  InitialCurrent=0  Capacitance=1e-6  Setx0=off  InitialVoltage=0  Measurements=None
  arm para1 : powerlib/Elements/Series RLC Branch  LConnTagsString=__new0  RConnTagsString=__new0  BranchType=RL  Resistance=R  Inductance=L  SetiL0=off  InitialCurrent=0  Capacitance=1e-6  Setx0=off  InitialVoltage=0  Measurements=None
  arm para2 : powerlib/Elements/Series RLC Branch  LConnTagsString=__new0  RConnTagsString=__new0  BranchType=RL  Resistance=R  Inductance=L  SetiL0=off  InitialCurrent=0  Capacitance=1e-6  Setx0=off  InitialVoltage=0  Measurements=None
  ila : powerlib/Measurements/Current Measurement  PhasorSimulation=off  OutputType=Complex  PSBequivalent=0
  ila1 : powerlib/Measurements/Current Measurement  PhasorSimulation=off  OutputType=Complex  PSBequivalent=0
  ila2 : powerlib/Measurements/Current Measurement  PhasorSimulation=off  OutputType=Complex  PSBequivalent=0
  iua : powerlib/Measurements/Current Measurement  PhasorSimulation=off  OutputType=Complex  PSBequivalent=0
  iua1 : powerlib/Measurements/Current Measurement  PhasorSimulation=off  OutputType=Complex  PSBequivalent=0
  iua2 : powerlib/Measurements/Current Measurement  PhasorSimulation=off  OutputType=Complex  PSBequivalent=0
  lower arm a : Subsystem
  lower arm b : Subsystem
  lower arm c : Subsystem
  upper arm a : Subsystem
  upper arm b : Subsystem
  upper arm c : Subsystem
  p : PMIOPort  Side=Right
  a : PMIOPort  Port=2  Side=Left
  b : PMIOPort  Port=3  Side=Left
  c : PMIOPort  Port=4  Side=Left
  n : PMIOPort  Port=5  Side=Right
  sigs : Outport
  wires:
  lower arm b/1(vc_lb) -> [vc_lb]
  [nlb] -> lower arm b/1(nlb)
  ila/1 -> [ila]
  [ila] -> lower arm a/2(ila)
  upper arm a/1(vc_ua) -> [vc_ua]
  lower arm a/1(vc_la) -> [vc_la]
  [ilb] -> lower arm b/2(ilb)
  [iua] -> upper arm a/2(iua)
  [nua] -> upper arm a/1(nua)
  [nub] -> upper arm b/1(nub)
  ila1/1 -> [ilb]
  [iub] -> upper arm b/2(iub)
  [nla] -> lower arm a/1(nla)
  upper arm b/1(vc_ub) -> [vc_ub]
  lower arm c/1(vc_lc) -> [vc_lc]
  [nlc] -> lower arm c/1(nlc)
  [iuc] -> upper arm c/2(iuc)
  [ilc] -> lower arm c/2(ilc)
  [nuc] -> upper arm c/1(nuc)
  ila2/1 -> [ilc]
  iua2/1 -> [iuc]
  upper arm c/1(vc_uc) -> [vc_uc]
  [vc_lc] -> Mux/12
  [vc_lb] -> Mux/11
  [vc_la] -> Mux/10
  [vc_uc] -> Mux/9
  [vc_ub] -> Mux/8
  [vc_ua] -> Mux/7
  [iua] -> Mux/1
  [iub] -> Mux/2
  [iuc] -> Mux/3
  [ila] -> Mux/4
  [ilb] -> Mux/5
  [ilc] -> Mux/6
  Mux/1 -> sigs/1
  iua/1 -> [iua]
  iua1/1 -> [iub]
  connections:
  upper arm b/LConn1 -- arm para1/LConn1
  ila/RConn1 -- lower arm a/RConn1
  ila/LConn1 -- arm para 2/RConn1
  ila1/LConn1 -- arm para 1/RConn1
  iua/RConn1 -- arm para 2/LConn1 -- a/RConn1
  iua1/RConn1 -- arm para 1/LConn1 -- b/RConn1
  iua1/LConn1 -- arm para1/RConn1
  ila1/RConn1 -- lower arm b/RConn1
  iua/LConn1 -- arm para/RConn1
  upper arm a/LConn1 -- arm para/LConn1
  ila2/RConn1 -- lower arm c/RConn1
  iua2/LConn1 -- arm para2/RConn1
  iua2/RConn1 -- arm para 3/LConn1 -- c/RConn1
  upper arm c/LConn1 -- arm para2/LConn1
  ila2/LConn1 -- arm para 3/RConn1
  lower arm c/LConn1 -- lower arm a/LConn1 -- lower arm b/LConn1 -- n/RConn1
  upper arm a/RConn1 -- upper arm c/RConn1 -- p/RConn1 -- upper arm b/RConn1

== system B2B_MMC/SM_MMC/RSS Grid/grid voltage ==
  Add : Sum  Inputs=+++
  Clock : Clock
  Constant : Constant  Value=-[0 2*pi/3 4*pi/3]
  Constant1 : Constant  Value=grid.phase
  Demux : Demux  Outputs=3
  Gain : Gain  Gain=w
  Gain1 : Gain  Gain=grid.va_peak
  Scope : Scope
  Trigonometric Function : Trigonometry
  cvs1 : powerlib/Electrical Sources/Controlled Voltage Source  Initialize=off  Source_Type=AC  Amplitude=0  Phase=0  Frequency=0  Measurements=None
  cvs2 : powerlib/Electrical Sources/Controlled Voltage Source  Initialize=off  Source_Type=AC  Amplitude=0  Phase=0  Frequency=0  Measurements=None
  cvs3 : powerlib/Electrical Sources/Controlled Voltage Source  Initialize=off  Source_Type=AC  Amplitude=0  Phase=0  Frequency=0  Measurements=None
  va_ph : PMIOPort  Side=Right
  vb_ph : PMIOPort  Port=2  Side=Right
  vc_ph : PMIOPort  Port=3  Side=Right
  wires:
  Demux/3 -> cvs3/1
  Demux/2 -> cvs2/1
  Constant1/1 -> Add/3
  Constant/1 -> Add/2
  Trigonometric Function/1 -> Gain1/1
  Demux/1 -> cvs1/1
  Gain/1 -> Add/1
  Clock/1 -> Gain/1
  Add/1 -> Trigonometric Function/1
  Gain1/1 -> Demux/1, Scope/1
  connections:
  cvs1/LConn1 -- cvs3/LConn1 -- cvs2/LConn1
  cvs3/RConn1 -- vc_ph/RConn1
  cvs2/RConn1 -- vb_ph/RConn1
  cvs1/RConn1 -- va_ph/RConn1

== system B2B_MMC/SM_MMC/SSS Grid/grid voltage ==
  Add : Sum  Inputs=+++
  Clock : Clock
  Constant : Constant  Value=-[0 2*pi/3 4*pi/3]
  Constant1 : Constant  Value=grid.phase
  Demux : Demux  Outputs=3
  Gain : Gain  Gain=w
  Gain1 : Gain  Gain=grid.va_peak
  Ground : powerlib/Elements/Ground  LConnTagsString=a
  Scope : Scope
  Trigonometric Function : Trigonometry
  cvs1 : powerlib/Electrical Sources/Controlled Voltage Source  Initialize=off  Source_Type=AC  Amplitude=0  Phase=0  Frequency=0  Measurements=None
  cvs2 : powerlib/Electrical Sources/Controlled Voltage Source  Initialize=off  Source_Type=AC  Amplitude=0  Phase=0  Frequency=0  Measurements=None
  cvs3 : powerlib/Electrical Sources/Controlled Voltage Source  Initialize=off  Source_Type=AC  Amplitude=0  Phase=0  Frequency=0  Measurements=None
  va_ph : PMIOPort  Side=Right
  vb_ph : PMIOPort  Port=2  Side=Right
  vc_ph : PMIOPort  Port=3  Side=Right
  wires:
  Demux/3 -> cvs3/1
  Demux/2 -> cvs2/1
  Constant1/1 -> Add/3
  Constant/1 -> Add/2
  Trigonometric Function/1 -> Gain1/1
  Demux/1 -> cvs1/1
  Gain/1 -> Add/1
  Clock/1 -> Gain/1
  Add/1 -> Trigonometric Function/1
  Gain1/1 -> Demux/1, Scope/1
  connections:
  cvs1/LConn1 -- Ground/LConn1 -- cvs3/LConn1 -- cvs2/LConn1
  cvs3/RConn1 -- vc_ph/RConn1
  cvs2/RConn1 -- vb_ph/RConn1
  cvs1/RConn1 -- va_ph/RConn1

== system B2B_MMC/SM_MMC/MMC1/Control Box MMC1/Capacitor Voltages ==
  Mux : Mux  Inputs=2
  Mux2 : Mux  Inputs=2
  Mux3 : Mux  Inputs=2
  Sum of Elements{,1..5} (6 alike) : Sum  Inputs=+
  sum_vca_ul : Outport
  sum_vcb_ul : Outport  Port=2
  sum_vcc_ul : Outport  Port=3
  wires:
  [vc_ua] -> Sum of Elements/1
  [vc_la] -> Sum of Elements1/1
  [vc_uc] -> Sum of Elements4/1
  [vc_lc] -> Sum of Elements5/1
  [vc_lb] -> Sum of Elements3/1
  [vc_ub] -> Sum of Elements2/1
  Mux2/1 -> sum_vcb_ul/1
  Sum of Elements4/1 -> Mux3/1
  Sum of Elements/1 -> Mux/1
  Sum of Elements3/1 -> Mux2/2
  Sum of Elements2/1 -> Mux2/1
  Mux/1 -> sum_vca_ul/1
  Mux3/1 -> sum_vcc_ul/1
  Sum of Elements1/1 -> Mux/2
  Sum of Elements5/1 -> Mux3/2

== system B2B_MMC/SM_MMC/MMC1/Control Box MMC1/Controllers ==
  is* : Inport
  vpcc_ab : Inport  Port=2
  is_ab : Inport  Port=3
  ic : Inport  Port=4
  Circulating Current and Arm Energy Controller : Subsystem
  PR Output Current Controller : Subsystem
  vs* : Outport
  vc* : Outport  Port=2
  wires:
  Circulating Current and Arm Energy Controller/1(vc*) -> vc*/1
  PR Output Current Controller/1(vs*) -> vs*/1
  is*/1 -> PR Output Current Controller/1(isAB*)
  ic/1 -> Circulating Current and Arm Energy Controller/1(Ic)
  is_ab/1 -> PR Output Current Controller/2(is_ab)
  vpcc_ab/1 -> PR Output Current Controller/3(vpcc_ab)

== system B2B_MMC/SM_MMC/MMC1/Control Box MMC1/Current Transforms ==
  Gain : Gain  Gain=0.5
  Sum : Sum  Inputs=|+-
  Sum1 : Sum  Inputs=|++
  is : Outport
  ic : Outport  Port=2
  wires:
  Gain/1 -> ic/1
  Sum1/1 -> Gain/1
  [iu] -> Sum1/1, Sum/1
  Sum/1 -> is/1
  [il] -> Sum/2, Sum1/2

== system B2B_MMC/SM_MMC/MMC1/Control Box MMC1/Insertion Indices (Direct Voltage Control) ==
  note: vs_ref
  note: vd/2
  note: vl_ref
  note: vu_ref
  note: vd/2
  note: vs_ref
  vs* : Inport
  vc* : Inport  Port=2
  Divide : Product  Inputs=*/
  Divide1 : Product  Inputs=*/
  Saturation1 : Saturate  UpperLimit=1  LowerLimit=0
  Saturation2 : Saturate  UpperLimit=1  LowerLimit=0
  Subsystem : Subsystem  Commented=on
  Sum1 : Sum  Inputs=|+-
  Sum2 : Sum  Inputs=|++
  vd : Constant  Value=vd_ref
  nu : Outport
  nl : Outport  Port=2
  wires:
  vc*/1 -> Sum2/1, Sum1/1
  Sum1/1 -> Divide/1
  vd/1 -> Divide/2, Divide1/2
  vs*/1 -> Sum1/2, Sum2/2
  Sum2/1 -> Divide1/1
  Divide/1 -> Saturation1/1
  Divide1/1 -> Saturation2/1
  Saturation1/1 -> nu/1
  Saturation2/1 -> nl/1

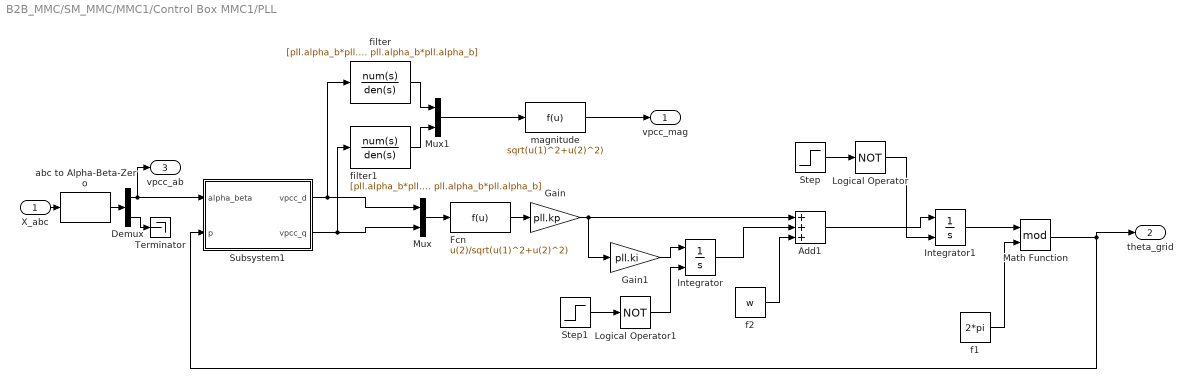
== system B2B_MMC/SM_MMC/MMC1/Control Box MMC1/PLL ==
  X_abc : Inport
  Add1 : Sum  Inputs=+++
  Demux : Demux  Outputs=2
  Fcn : Fcn  Expr=u(2)/sqrt(u(1)^2+u(2)^2)
  Gain : Gain  Gain=pll.kp
  Gain1 : Gain  Gain=pll.ki
  Integrator : Integrator  ExternalReset=level
  Integrator1 : Integrator  ExternalReset=level  InitialCondition=w
  Logical Operator : Logic  Operator=NOT  AllPortsSameDT=off  OutDataTypeStr=boolean
  Logical Operator1 : Logic  Operator=NOT  AllPortsSameDT=off  OutDataTypeStr=boolean
  Math Function : Math  Operator=mod  SaturateOnIntegerOverflow=on
  Mux : Mux  Inputs=2
  Mux1 : Mux  Inputs=2
  Step : Step  Time=1e-6  After=grid.enable  SampleTime=0
  Step1 : Step  Time=1e-6  After=grid.enable  SampleTime=0
  Subsystem1 : Subsystem
  Terminator : Terminator
  abc to Alpha-Beta-Zero : powerlib_meascontrol/Transformations/abc to Alpha-Beta-Zero
      settings: SourceProductName=Simscape Power Systems
  f1 : Constant  Value=2*pi
  f2 : Constant  Value=w
  filter : TransferFcn  Numerator=[pll.alpha_b*pll.alpha_b]  Denominator=[1 sqrt(2)*pll.alpha_b pll.alpha_b*pll.alpha_b]
  filter1 : TransferFcn  Numerator=[pll.alpha_b*pll.alpha_b]  Denominator=[1 sqrt(2)*pll.alpha_b pll.alpha_b*pll.alpha_b]
  magnitude : Fcn  Expr=sqrt(u(1)^2+u(2)^2)
  vpcc_mag : Outport
  theta_grid : Outport  Port=2
  vpcc_ab : Outport  Port=3
  wires:
  Add1/1 -> Integrator1/1
  Fcn/1 -> Gain/1
  Gain1/1 -> Integrator/1
  Gain/1 -> Add1/1, Gain1/1
  Integrator/1 -> Add1/2
  f2/1 -> Add1/3
  Integrator1/1 -> Math Function/1
  f1/1 -> Math Function/2
  Math Function/1 -> theta_grid/1, Subsystem1/2(p)
  Logical Operator1/1 -> Integrator/2
  Logical Operator/1 -> Integrator1/2
  Step1/1 -> Logical Operator1/1
  Demux/1 -> Subsystem1/1(alpha_beta), vpcc_ab/1
  abc to Alpha-Beta-Zero/1 -> Demux/1
  X_abc/1 -> abc to Alpha-Beta-Zero/1
  Demux/2 -> Terminator/1
  Mux/1 -> Fcn/1
  magnitude/1 -> vpcc_mag/1
  Subsystem1/2(vpcc_q) -> filter1/1, Mux/2
  Subsystem1/1(vpcc_d) -> Mux/1, filter/1
  filter/1 -> Mux1/1
  filter1/1 -> Mux1/2
  Mux1/1 -> magnitude/1
  Step/1 -> Logical Operator/1

== system B2B_MMC/SM_MMC/MMC1/Control Box MMC1/Reference Powers ==
  Product : Product
  Product1 : Product
  Product2 : Product
  Trigonometric Function : Trigonometry  Operator=cos
  Trigonometric Function1 : Trigonometry
  percentage loading : Constant  Value=load.percent
  percentage loading1 : Constant  Value=load.phi
  rated converter apparent power : Constant  Value=Smax
  p* : Outport
  q* : Outport  Port=2
  wires:
  rated converter apparent power/1 -> Product/1
  percentage loading/1 -> Product/2
  percentage loading1/1 -> Trigonometric Function/1, Trigonometric Function1/1
  Trigonometric Function/1 -> Product1/1
  Product/1 -> Product2/1, Product1/2
  Trigonometric Function1/1 -> Product2/2
  Product2/1 -> q*/1
  Product1/1 -> p*/1

== system B2B_MMC/SM_MMC/MMC1/Control Box MMC1/Subsystem ==
  vpcc : Inport
  is_meas : Inport  Port=2
  Demux{,1..3} (4 alike) : Demux  Outputs=3
  Fcn : Fcn  Expr=(u(1)*u(4)) + (u(2)*u(5)) + (u(3)*u(6))
  Fcn1 : Fcn  Expr="( (u(1)-u(2))*u(6) +  (u(3)-u(1))*u(5)  + (u(2)-u(3))*u(4) )/sqrt(3)"
  Mux1 : Mux  Inputs=2
  Mux2 : Mux  Inputs=2
  Mux3 : Mux  Inputs=6
  Transfer Fcn : TransferFcn  Numerator=[2*pi*5]  Denominator=[1 2*pi*5]
  Transfer Fcn1 : TransferFcn  Numerator=[2*pi*5]  Denominator=[1 2*pi*5]
  vs : Outport
  is : Outport  Port=2
  meas_p : Outport  Port=3
  meas_q : Outport  Port=4
  wires:
  Demux/1 -> Mux3/1, Mux2/1
  Demux3/1 -> Mux2/2
  [vsref_abc] -> Demux3/1
  Demux2/1 -> Mux1/2
  Demux1/1 -> Mux3/4, Mux1/1
  Mux2/1 -> vs/1
  vpcc/1 -> Demux/1
  is_meas/1 -> Demux1/1
  Mux1/1 -> is/1
  [isref_abc] -> Demux2/1
  Fcn/1 -> Transfer Fcn/1
  Demux/2 -> Mux3/2
  Demux/3 -> Mux3/3
  Mux3/1 -> Fcn1/1, Fcn/1
  Demux1/2 -> Mux3/5
  Demux1/3 -> Mux3/6
  Transfer Fcn/1 -> meas_p/1
  Transfer Fcn1/1 -> meas_q/1
  Fcn1/1 -> Transfer Fcn1/1

== system B2B_MMC/SM_MMC/MMC1/Control Box MMC1/Transform1 ==
  is : Inport
  Demux : Demux  Outputs=2
  Terminator : Terminator
  abc to Alpha-Beta-Zero : powerlib_meascontrol/Transformations/abc to Alpha-Beta-Zero
      settings: SourceProductName=Simscape Power Systems
  is_ab : Outport
  wires:
  is/1 -> abc to Alpha-Beta-Zero/1
  abc to Alpha-Beta-Zero/1 -> Demux/1
  Demux/1 -> is_ab/1
  Demux/2 -> Terminator/1

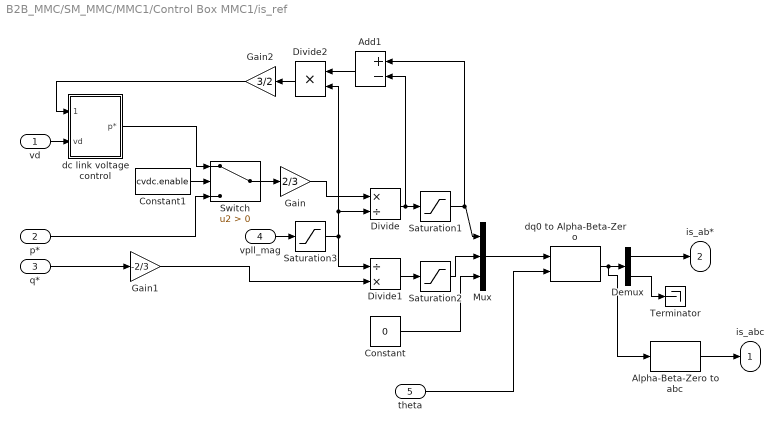
== system B2B_MMC/SM_MMC/MMC1/Control Box MMC1/is_ref ==
  vd : Inport
  p* : Inport  Port=2
  q* : Inport  Port=3
  vpll_mag : Inport  Port=4
  theta : Inport  Port=5
  Add1 : Sum  Inputs=+-
  Alpha-Beta-Zero to abc : powerlib_meascontrol/Transformations/Alpha-Beta-Zero to abc
      settings: SourceProductName=Simscape Power Systems  SourceProductBaseCode=PS
  Constant : Constant  Value=0
  Constant1 : Constant  Value=cvdc.enable
  Demux : Demux  Outputs=2
  Divide : Product  Inputs=*/
  Divide1 : Product  Inputs=/*
  Divide2 : Product  Inputs=**
  Gain : Gain  Gain=2/3
  Gain1 : Gain  Gain=-2/3
  Gain2 : Gain  Gain=3/2
  Mux : Mux  Inputs=3
  Saturation1 : Saturate  UpperLimit=is_max  LowerLimit=-is_max
  Saturation2 : Saturate  UpperLimit=is_max  LowerLimit=-is_max
  Saturation3 : Saturate  UpperLimit=1e9  LowerLimit=1e-6
  Switch : Switch  Criteria=u2 > Threshold
  Terminator : Terminator
  dc link voltage control : Subsystem
  dq0 to Alpha-Beta-Zero : powerlib_meascontrol/Transformations/dq0 to Alpha-Beta-Zero  Alignment=Aligned with phase A axis
      settings: SourceProductName=Simscape Power Systems  SourceProductBaseCode=PS
  is_abc : Outport
  is_ab* : Outport  Port=2
  wires:
  q*/1 -> Gain1/1
  Gain/1 -> Divide/1
  Saturation3/1 -> Divide/2, Divide2/2, Divide1/1
  Gain1/1 -> Divide1/2
  Constant/1 -> Mux/3
  Mux/1 -> dq0 to Alpha-Beta-Zero/1
  dq0 to Alpha-Beta-Zero/1 -> Alpha-Beta-Zero to abc/1, Demux/1
  Demux/2 -> Terminator/1
  Demux/1 -> is_ab*/1
  theta/1 -> dq0 to Alpha-Beta-Zero/2
  Divide/1 -> Add1/2, Saturation1/1
  Saturation1/1 -> Add1/1, Mux/1
  Divide1/1 -> Saturation2/1
  Saturation2/1 -> Mux/2
  vpll_mag/1 -> Saturation3/1
  Alpha-Beta-Zero to abc/1 -> is_abc/1
  vd/1 -> dc link voltage control/2(vd)
  Add1/1 -> Divide2/1
  Divide2/1 -> Gain2/1
  Gain2/1 -> dc link voltage control/1(antiwp)
  Switch/1 -> Gain/1
  dc link voltage control/1(p*) -> Switch/1
  p*/1 -> Switch/3
  Constant1/1 -> Switch/2
